simulink model "Model_extended_estimator_bb"  (R2024b)
settings: Solver=VariableStepAuto  StartTime=0.0  StopTime=4  RelTol=1e-3
values from neighbouring files (symbols this model uses):
  Ae = [A_rho zeros(3,2); B_c*C_rho A_c]    [Controller_StateSpace_Lab1_25_04_25.m]
  Be = [0; 0; 0; B_c]    [Controller_StateSpace_Lab1_25_04_25.m]
  C_rho = [1 0 0]    [Controller_StateSpace_Lab1_25_04_25.m]
  Ce = [0 0 0 C_c]    [Controller_StateSpace_Lab1_25_04_25.m]
  K_stateFB_extended = place(A_c, B_c, p)    [Controller_StateSpace_Lab1_25_04_25.m]
  Le = L_transpose'    [Controller_StateSpace_Lab1_25_04_25.m]
undefined symbols (not defined in the file or in its folder): pulse2deg, rads2rpm
settings Model: Creator=Riccardo Grosso  LastModifiedBy=Buton

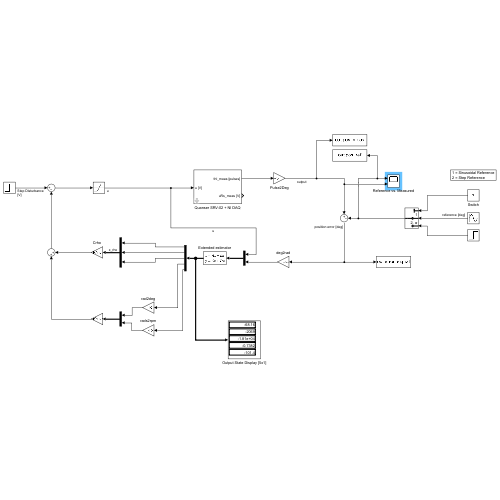
[thumbnail: Simulink's stored preview of the top-level diagram]
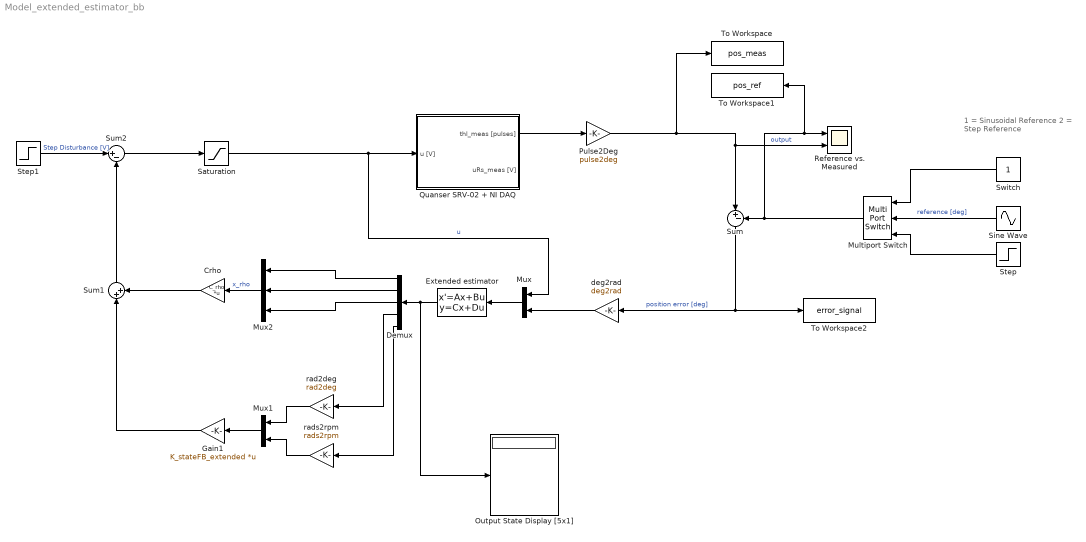
== system Model_extended_estimator_bb ==
  note: 1 = Sinusoidal Reference
      | 2 = Step Reference
  Crho : Gain  Gain=C_rho  Multiplication=Matrix(K*u) (u vector)
  Demux : Demux  Outputs=5
  Extended estimator : StateSpace  A=Ae-Le*Ce  B=[Be Le]  C=eye(5,5)  D=zeros(5,2)  InitialCondition=0
  Gain1 : Gain  Gain=K_stateFB_extended  Multiplication=Matrix(K*u) (u vector)
  Multiport Switch : MultiPortSwitch  Inputs=2  SaturateOnIntegerOverflow=off  InputSameDT=off
  Mux : Mux  Inputs=2
  Mux1 : Mux  Inputs=2
  Mux2 : Mux  Inputs=3
  Output State Display [5x1] : Display
  Pulse2Deg : Gain  Gain=pulse2deg
  Quanser SRV-02 + NI DAQ : Subsystem  mask(Quanser SRV-02 (with inertial load) + NI DAQ){Ts=0.001, fricType=Karnopp}
      mask prompts: Ts "NI DAQ Sample Time:"; fricType "Friction model"
      mask help: Quanser SRV-02 (with inertial load) + NI DAQ model.
      mask init:
      | %%  Sensors data
      | 
      | %   shunt resistor
      | sens.curr.Rs = 0.5;                         %   resistance [Ohm]   
      | sens.curr.uRs_std = 0.01;                   %   voltage noise standard dev [V]                           
      | sens.curr.uRs_var = sens.curr.uRs_std^2;	%   voltage noise variance [V^2]
      | 
      | %   Hewlett-Packard HEDS-5540#A06 optical encoder
      | sens.enc.ppr = 500*4;                       %   pulses per rotation
      | sens.enc.pulse2deg = 360/sens.enc.ppr;      %   [pulses] -> [deg]
      | sens.enc.pulse2rad = 2*pi/sens.enc.ppr;     %   [pulses] -> [rad]
      | sens.enc.deg2pulse = sens.enc.ppr/360;      %   [deg] -> [pulses]
      | sens.enc.rad2pulse = sens.enc.ppr/2/pi;     %   [rad] -> [pulses]
      | 
      | 
      | %%  Data acquisition board (daq) data
      | 
      | %   NI PCI-6221 DAC data
      | daq.dac.bits = 16;                                  %   resolution (bits)
      | daq.dac.fs   = 10;                                  %   full scale 
      | daq.dac.q    = 2*daq.dac.fs/(2^daq.dac.bits-1);     %	quantization
      | 
      | %   NI PCI-6221 ADC data
      | daq.adc.bits = 16;                                  %   resolution (bits)
      | daq.adc.fs   = 10;                                  %   full scale (as set in SLDRT Analog Input block)
      | daq.adc.q    = 2*daq.adc.fs/(2^daq.adc.bits-1);     %   quantization
      mask Help:
      | Riccardo Antonello (antonello@dei.unipd.it)
      | 
      | April 24, 2020
      | 
      | Dept. of Information Engineering, University of Padova
      mask TypeOptions fricType: Coulomb + viscous | Karnopp
  Reference vs. Measured : Scope  NumInputPorts=2
  Saturation : Saturate  UpperLimit=12  LowerLimit=-12  ZeroCross=off
  Sine Wave : Sin  Amplitude=40  Frequency=2*pi*(1/0.1)  SampleTime=0
  Step : Step  Time=0  After=40  SampleTime=0
  Step1 : Step  Time=0  After=2  SampleTime=0
  Sum : Sum  Inputs=|+-
  Sum1 : Sum  Inputs=|++
  Sum2 : Sum  Inputs=|+-
  Switch : Constant
  To Workspace : ToWorkspace  VariableName=pos_meas  SaveFormat=Timeseries  SampleTime=-1
  To Workspace1 : ToWorkspace  VariableName=pos_ref  SaveFormat=Timeseries  SampleTime=-1
  To Workspace2 : ToWorkspace  VariableName=error_signal  SaveFormat=Timeseries  SampleTime=-1
  deg2rad : Gain  Gain=deg2rad
  rad2deg : Gain  Gain=rad2deg
  rads2rpm : Gain  Gain=rads2rpm
  wires:
  Mux1/1 -> Gain1/1
  Crho/1 -> Sum1/2
  Gain1/1 -> Sum1/1
  Sum1/1 -> Sum2/2
  Quanser SRV-02 + NI DAQ/1(thl_meas [pulses]) -> Pulse2Deg/1
  Pulse2Deg/1 -> To Workspace/1, Reference vs. Measured/2, Sum/1  "output"
  Mux/1 -> Extended estimator/1
  deg2rad/1 -> Mux/2
  Sum/1 -> To Workspace2/1, deg2rad/1  "position error [deg]"
  rad2deg/1 -> Mux1/1
  rads2rpm/1 -> Mux1/2
  Sum2/1 -> Saturation/1
  Saturation/1 -> Mux/1, Quanser SRV-02 + NI DAQ/1(u [V])  "u"
  Mux2/1 -> Crho/1  "x_rho"
  Extended estimator/1 -> Output State Display [5x1]/1, Demux/1
  Demux/1 -> Mux2/1
  Demux/2 -> Mux2/2
  Demux/3 -> Mux2/3
  Demux/4 -> rad2deg/1
  Demux/5 -> rads2rpm/1
  Step1/1 -> Sum2/1  "Step Disturbance [V]"
  Multiport Switch/1 -> To Workspace1/1, Reference vs. Measured/1, Sum/2
  Sine Wave/1 -> Multiport Switch/2  "reference [deg]"
  Step/1 -> Multiport Switch/3
  Switch/1 -> Multiport Switch/1

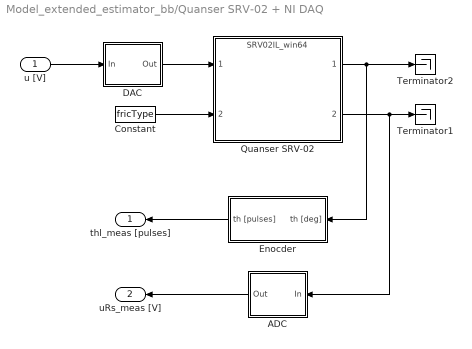
== system Model_extended_estimator_bb/Quanser SRV-02 + NI DAQ ==
  u [V] : Inport
  ADC : Subsystem
  Constant : Constant  Value=fricType
  DAC : Subsystem
  Enocder : Subsystem
  Quanser SRV-02 : ModelReference  ModelNameDialog=SRV02IL_win64.slxp  ModelReferenceVersion=1.44  CopyOfModelProtected=on
  Terminator1 : Terminator
  Terminator2 : Terminator
  thl_meas [pulses] : Outport
  uRs_meas [V] : Outport  Port=2
  wires:
  Enocder/1(th [pulses]) -> thl_meas [pulses]/1
  ADC/1(Out) -> uRs_meas [V]/1
  DAC/1(Out) -> Quanser SRV-02/1
  Quanser SRV-02/2 -> ADC/1(In), Terminator1/1
  u [V]/1 -> DAC/1(In)
  Quanser SRV-02/1 -> Enocder/1(th [deg]), Terminator2/1
  Constant/1 -> Quanser SRV-02/2

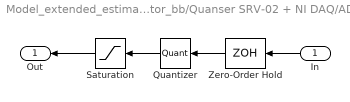
== system Model_extended_estimator_bb/Quanser SRV-02 + NI DAQ/ADC ==
  In : Inport
  Quantizer : Quantizer  QuantizationInterval=daq.adc.q
  Saturation : Saturate  UpperLimit=daq.adc.fs  LowerLimit=-daq.adc.fs
  Zero-Order Hold : ZeroOrderHold  SampleTime=Ts
  Out : Outport
  wires:
  Saturation/1 -> Out/1
  In/1 -> Zero-Order Hold/1
  Quantizer/1 -> Saturation/1
  Zero-Order Hold/1 -> Quantizer/1

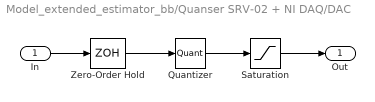
== system Model_extended_estimator_bb/Quanser SRV-02 + NI DAQ/DAC ==
  In : Inport
  Quantizer : Quantizer  QuantizationInterval=daq.dac.q
  Saturation : Saturate  UpperLimit=daq.dac.fs  LowerLimit=-daq.dac.fs
  Zero-Order Hold : ZeroOrderHold  SampleTime=Ts
  Out : Outport
  wires:
  Quantizer/1 -> Saturation/1
  In/1 -> Zero-Order Hold/1
  Zero-Order Hold/1 -> Quantizer/1
  Saturation/1 -> Out/1

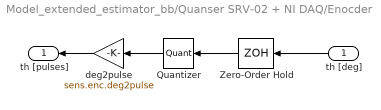
== system Model_extended_estimator_bb/Quanser SRV-02 + NI DAQ/Enocder ==
  th [deg] : Inport
  Quantizer : Quantizer  QuantizationInterval=sens.enc.pulse2deg
  Zero-Order Hold : ZeroOrderHold  SampleTime=Ts
  deg2pulse : Gain  Gain=sens.enc.deg2pulse
  th [pulses] : Outport
  wires:
  Quantizer/1 -> deg2pulse/1
  th [deg]/1 -> Zero-Order Hold/1
  Zero-Order Hold/1 -> Quantizer/1
  deg2pulse/1 -> th [pulses]/1
